simulink model "RZ_DAC"  (Simulink 7.9)
settings: Solver=ode45  StartTime=0.0  StopTime=simu.trantime  RelTol=1e-3
undefined symbols (not defined in the file): Fs
settings Model: Creator=amyles  LastModifiedBy=Arnaldi Isacco
settings SolverCC: ZeroCrossAlgorithm=Adaptive  AutoInsertRateTranBlk=on
settings DataIOCC: MaxDataPoints=50000  SaveOutput=off  SaveTime=off
settings OptimizationCC: InlineParams=on
settings DebuggingCC: UnderspecifiedInitializationDetection=Simplified  InvalidFcnCallConnMsg=none  StrictBusMsg=ErrorOnBusTreatedAsVector
settings ModelReferenceCC: ModelReferenceNumInstancesAllowed=Single
settings CodeAppCC: CustomSymbolStrType=$N$R$M_T
settings GRTTargetCC: CombineOutputUpdateFcns=off  GRTInterface=on

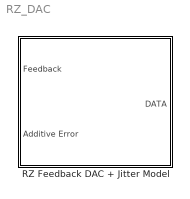
== system RZ_DAC ==
  RZ Feedback DAC + Jitter Model : Subsystem

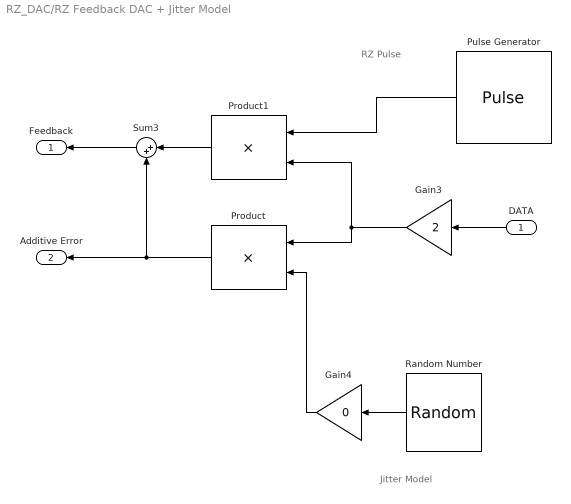
== system RZ_DAC/RZ Feedback DAC + Jitter Model ==
  note: Jitter Model
  note: RZ Pulse
  DATA : Inport
  Gain3 : Gain  Gain=2  SampleTime=1/Fs
  Gain4 : Gain  Gain=0  SampleTime=1/Fs
  Product : Product  SampleTime=1/Fs  RndMeth=Zero
  Product1 : Product  SampleTime=1/Fs  RndMeth=Zero
  Pulse Generator : DiscretePulseGenerator  PulseType=Time based  Amplitude=0.5  Period=1/Fs  PulseWidth=25  SampleTime=1/Fs
  Random Number : RandomNumber  Mean=100e-12  Variance=50e-9  Seed=1  SampleTime=1/Fs
  Sum3 : Sum  Inputs=|++  SampleTime=1/Fs
  Feedback : Outport
  Additive Error : Outport  Port=2
  wires:
  DATA/1 -> Gain3/1
  Pulse Generator/1 -> Product1/1
  Gain3/1 -> Product1/2, Product/1
  Random Number/1 -> Gain4/1
  Gain4/1 -> Product/2
  Product/1 -> Sum3/2, Additive Error/1
  Product1/1 -> Sum3/1
  Sum3/1 -> Feedback/1
